simulink model "Dcmotor_new"  (R2024b)
settings: Solver=ode23t  StartTime=0.0  StopTime=10.0  FixedStep=0.001  MaxStep=0.001  MinStep=1e-8  RelTol=1e-4  AbsTol=1e-4
InitFcn:
  | clear
  | clc
  | 
  | J=0.02;
  | b=0.1;
  | Ke=0.05;
  | Kt=0.05;
  | R=1;
  | L=0.01;
settings Model: Creator=lenovo  LastModifiedBy=girija
settings SolverCC: MaxConsecutiveMinStep=10
settings OptimizationCC: ReuseModelBlockBuffer=off
settings RTWCC: GPUComputeCapability=3.5

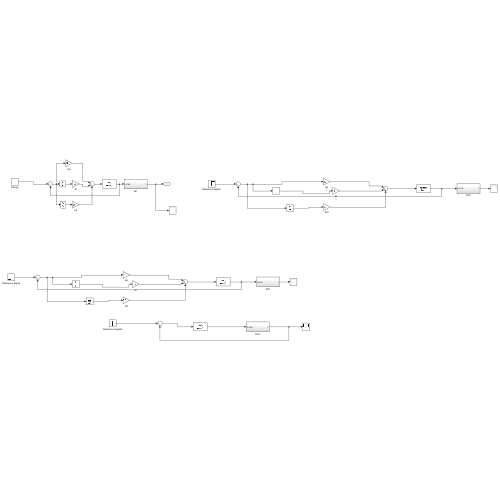
[thumbnail: Simulink's stored preview of the top-level diagram]
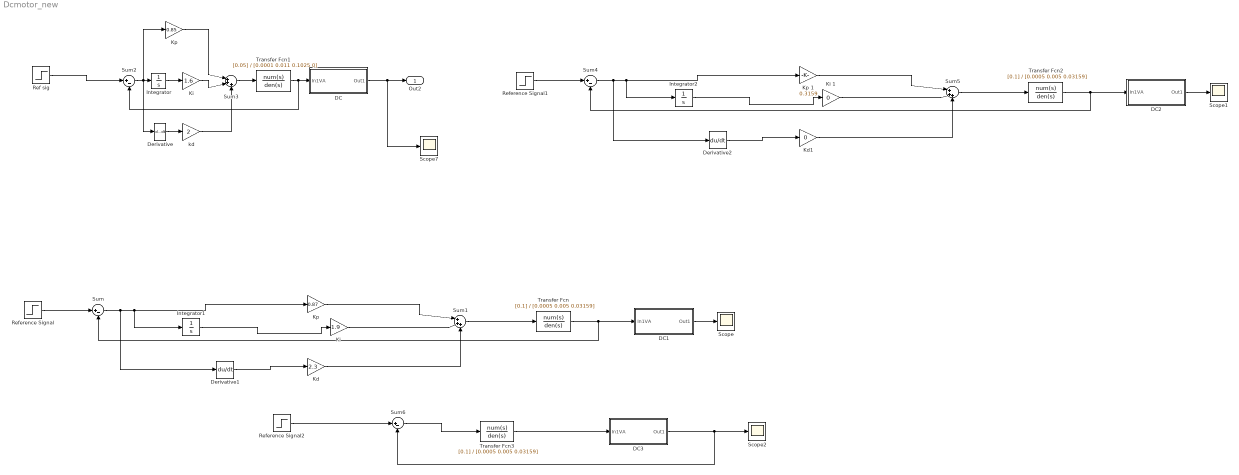
== system Dcmotor_new ==
  DC : Subsystem
  DC1 : Subsystem
  DC2 : Subsystem
  DC3 : Subsystem
  Derivative : Derivative
  Derivative1 : Derivative
  Derivative2 : Derivative
  Integrator : Integrator
  Integrator1 : Integrator
  Integrator2 : Integrator
  Kd : Gain  Gain=2.3
  Kd1 : Gain  Gain=0
  Ki : Gain  Gain=1.6
  "Ki " : Gain  Gain=1.9
  Ki 1 : Gain  Gain=0
  Kp : Gain  Gain=0.85
  "Kp " : Gain  Gain=0.87
  Kp 1 : Gain  Gain=0.3159
  Ref sig : Step  SampleTime=0
  Reference Signal : Step  SampleTime=0
  Reference Signal1 : Step  SampleTime=0
  Reference Signal2 : Step  SampleTime=0
  Scope{,1..2,7} (4 alike) : Scope
  Sum{,2,4,6} (4 alike) : Sum  Inputs=|+-
  Sum1 : Sum  Inputs=|+++
  Sum3 : Sum  Inputs=|+++
  Sum5 : Sum  Inputs=|+++
  Transfer Fcn : TransferFcn  Numerator=[0.1]  Denominator=[0.0005 0.005 0.03159]
  Transfer Fcn1 : TransferFcn  Numerator=[0.05]  Denominator=[0.0001 0.011 0.1025 0]
  Transfer Fcn2 : TransferFcn  Numerator=[0.1]  Denominator=[0.0005 0.005 0.03159]
  Transfer Fcn3 : TransferFcn  Numerator=[0.1]  Denominator=[0.0005 0.005 0.03159]
  kd : Gain  Gain=2
  Out2 : Outport
  wires:
  Kp/1 -> Sum3/1
  Ki/1 -> Sum3/2
  kd/1 -> Sum3/3
  DC/1(Out1) -> Scope7/1, Out2/1
  Sum2/1 -> Kp/1, Integrator/1, Derivative/1
  Derivative/1 -> kd/1
  Integrator/1 -> Ki/1
  Transfer Fcn/1 -> DC1/1(In1VA), Sum/2
  Sum1/1 -> Transfer Fcn/1
  Reference Signal/1 -> Sum/1
  "Ki "/1 -> Sum1/2
  Kd/1 -> Sum1/3
  "Kp "/1 -> Sum1/1
  Sum3/1 -> Transfer Fcn1/1
  Transfer Fcn1/1 -> Sum2/2, DC/1(In1VA)
  Sum/1 -> Derivative1/1, Integrator1/1, "Kp "/1
  Integrator1/1 -> "Ki "/1
  Derivative1/1 -> Kd/1
  DC1/1(Out1) -> Scope/1
  Ref sig/1 -> Sum2/1
  DC2/1(Out1) -> Scope1/1
  Sum4/1 -> Derivative2/1, Integrator2/1, Kp 1/1
  Kp 1/1 -> Sum5/1
  Kd1/1 -> Sum5/3
  Ki 1/1 -> Sum5/2
  Reference Signal1/1 -> Sum4/1
  Derivative2/1 -> Kd1/1
  Sum5/1 -> Transfer Fcn2/1
  Integrator2/1 -> Ki 1/1
  Transfer Fcn2/1 -> DC2/1(In1VA), Sum4/2
  Reference Signal2/1 -> Sum6/1
  Sum6/1 -> Transfer Fcn3/1
  Transfer Fcn3/1 -> DC3/1(In1VA)
  DC3/1(Out1) -> Sum6/2, Scope2/1

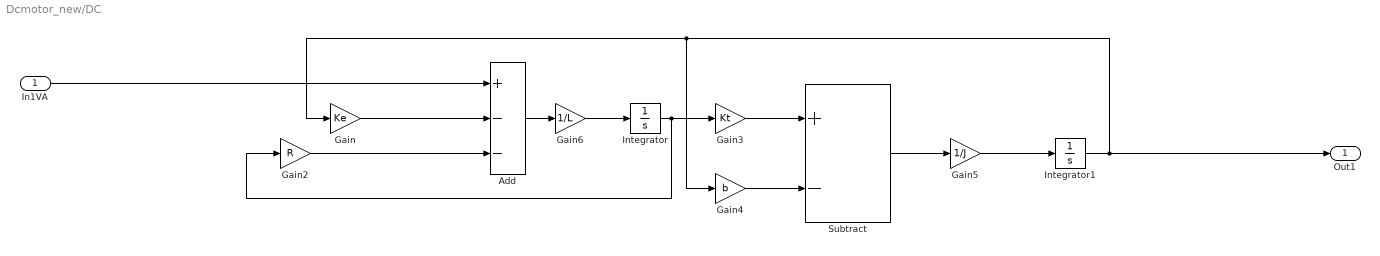
== system Dcmotor_new/DC ==
  In1VA : Inport
  Add : Sum  Inputs=+--
  Gain : Gain  Gain=Ke
  Gain2 : Gain  Gain=R
  Gain3 : Gain  Gain=Kt
  Gain4 : Gain  Gain=b
  Gain5 : Gain  Gain=1/J
  Gain6 : Gain  Gain=1/L
  Integrator : Integrator
  Integrator1 : Integrator
  Subtract : Sum  Inputs=+-
  Out1 : Outport
  wires:
  Integrator1/1 -> Out1/1, Gain4/1, Gain/1
  Integrator/1 -> Gain2/1, Gain3/1
  Gain2/1 -> Add/3
  Add/1 -> Gain6/1
  Gain5/1 -> Integrator1/1
  Gain3/1 -> Subtract/1
  In1VA/1 -> Add/1
  Gain6/1 -> Integrator/1
  Gain4/1 -> Subtract/2
  Gain/1 -> Add/2
  Subtract/1 -> Gain5/1

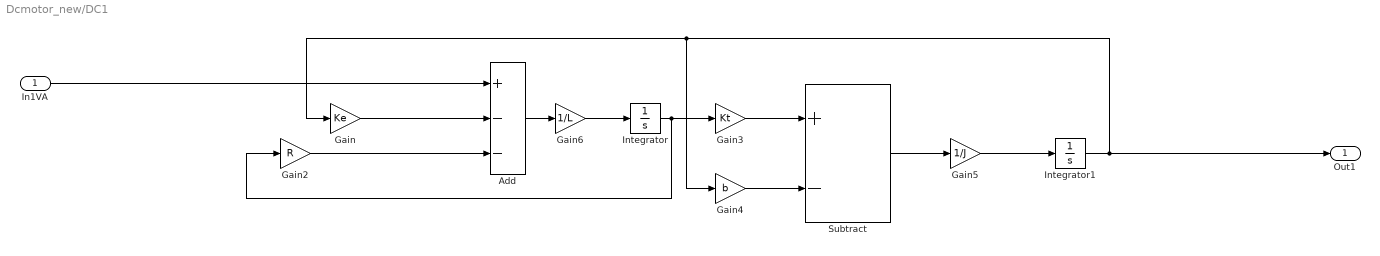
== system Dcmotor_new/DC1 ==
  In1VA : Inport
  Add : Sum  Inputs=+--
  Gain : Gain  Gain=Ke
  Gain2 : Gain  Gain=R
  Gain3 : Gain  Gain=Kt
  Gain4 : Gain  Gain=b
  Gain5 : Gain  Gain=1/J
  Gain6 : Gain  Gain=1/L
  Integrator : Integrator
  Integrator1 : Integrator
  Subtract : Sum  Inputs=+-
  Out1 : Outport
  wires:
  Integrator1/1 -> Out1/1, Gain4/1, Gain/1
  Integrator/1 -> Gain2/1, Gain3/1
  Gain2/1 -> Add/3
  Add/1 -> Gain6/1
  Gain5/1 -> Integrator1/1
  Gain3/1 -> Subtract/1
  In1VA/1 -> Add/1
  Gain6/1 -> Integrator/1
  Gain4/1 -> Subtract/2
  Gain/1 -> Add/2
  Subtract/1 -> Gain5/1

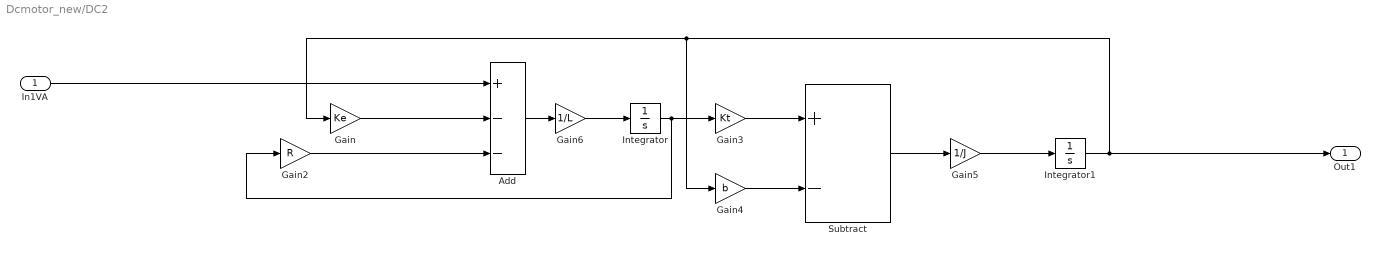
== system Dcmotor_new/DC2 ==
  In1VA : Inport
  Add : Sum  Inputs=+--
  Gain : Gain  Gain=Ke
  Gain2 : Gain  Gain=R
  Gain3 : Gain  Gain=Kt
  Gain4 : Gain  Gain=b
  Gain5 : Gain  Gain=1/J
  Gain6 : Gain  Gain=1/L
  Integrator : Integrator
  Integrator1 : Integrator
  Subtract : Sum  Inputs=+-
  Out1 : Outport
  wires:
  Integrator1/1 -> Out1/1, Gain4/1, Gain/1
  Integrator/1 -> Gain2/1, Gain3/1
  Gain2/1 -> Add/3
  Add/1 -> Gain6/1
  Gain5/1 -> Integrator1/1
  Gain3/1 -> Subtract/1
  In1VA/1 -> Add/1
  Gain6/1 -> Integrator/1
  Gain4/1 -> Subtract/2
  Gain/1 -> Add/2
  Subtract/1 -> Gain5/1

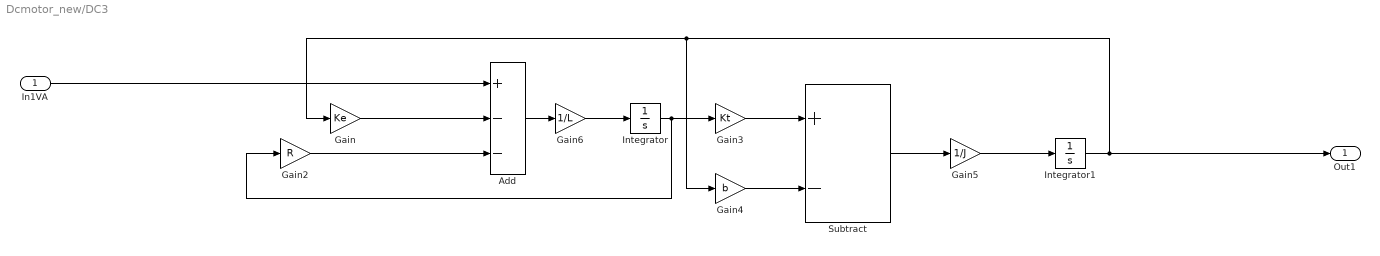
== system Dcmotor_new/DC3 ==
  In1VA : Inport
  Add : Sum  Inputs=+--
  Gain : Gain  Gain=Ke
  Gain2 : Gain  Gain=R
  Gain3 : Gain  Gain=Kt
  Gain4 : Gain  Gain=b
  Gain5 : Gain  Gain=1/J
  Gain6 : Gain  Gain=1/L
  Integrator : Integrator
  Integrator1 : Integrator
  Subtract : Sum  Inputs=+-
  Out1 : Outport
  wires:
  Integrator1/1 -> Out1/1, Gain4/1, Gain/1
  Integrator/1 -> Gain2/1, Gain3/1
  Gain2/1 -> Add/3
  Add/1 -> Gain6/1
  Gain5/1 -> Integrator1/1
  Gain3/1 -> Subtract/1
  In1VA/1 -> Add/1
  Gain6/1 -> Integrator/1
  Gain4/1 -> Subtract/2
  Gain/1 -> Add/2
  Subtract/1 -> Gain5/1
